simulink model "fundamentalModel"  (R2023a)
settings: Solver=FixedStepAuto  StartTime=0.0  StopTime=1681200  FixedStep=60  RelTol=1e-3
model workspace (MAT data in the model file):
  c1 = Simulink.Parameter
  c1.Value = Simulink.data.Expression
  c1.Value.ExpressionString = " rho_s/rho_m"
  c1.DataType = 'auto'
  c1.Complexity = 'real'
  c1.Dimensions = -1
  c2 = Simulink.Parameter
  c2.Value = Simulink.data.Expression
  c2.Value.ExpressionString = " 1/(rho_m*pi*R^2)"
  c2.DataType = 'auto'
  c2.Complexity = 'real'
  c2.Dimensions = -1
  c3 = Simulink.Parameter
  c3.Value = Simulink.data.Expression
  c3.Value.ExpressionString = " r_m^2*(2*g)^0.5/(R^2)"
  c3.DataType = 'auto'
  c3.Complexity = 'real'
  c3.Dimensions = -1
  c4 = Simulink.Parameter
  c4.Value = Simulink.data.Expression
  c4.Value.ExpressionString = " 1/(rho_m*Cp_matte)"
  c4.DataType = 'auto'
  c4.Complexity = 'real'
  c4.Dimensions = -1
  c5 = Simulink.Parameter
  c5.Value = Simulink.data.Expression
  c5.Value.ExpressionString = " r_s^2*(2*g)^0.5/(R^2)"
  c5.DataType = 'auto'
  c5.Complexity = 'real'
  c5.Dimensions = -1
undefined symbols (not defined in the file or in its folder): a, alpha_Co, alpha_Cu, alpha_Fe, alpha_Ni, b, Cp_bar_eq, Cp_bar_offgas, Cp_bar_slag, Cp_matte, Cp_slag, delta_H_bar_r_coal, delta_H_CoS, delta_H_Cu2S, delta_H_FeS, delta_H_Ni3S2, delta_Ts, epsilon, g, hm_init, hs_hole, m_dot_dust_and_accr, R, r_m, r_s, rho_m, rho_s, sigma, T_amb, T_furnace, Tm_init, U, vFactor_m, vFactor_s
libraries: simulink x3
settings Model: PauseTimes=1.631410e4  PacingRate=1000  Creator=jason.miskin  LastModifiedBy=john.atherfold
settings DataIOCC: ExternalInput=slInputs  LoadExternalInput=on  SaveFormat=Array  InspectSignalLogs=on  OutputOption=AdditionalOutputTimes  OutputTimes=SDO_OutputTimes  ReturnWorkspaceOutputsName=SDOSimTest_Log
settings DebuggingCC: UnconnectedInputMsg=warning  UnconnectedOutputMsg=warning  UnconnectedLineMsg=warning
settings ModelReferenceCC: EnableRefExpFcnMdlSchedulingChecks=on
settings RTWCC: DLArmComputeVersion=19.05

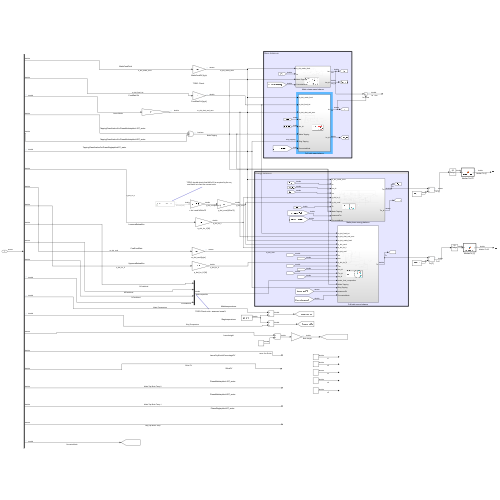
[thumbnail: Simulink's stored preview of the top-level diagram]
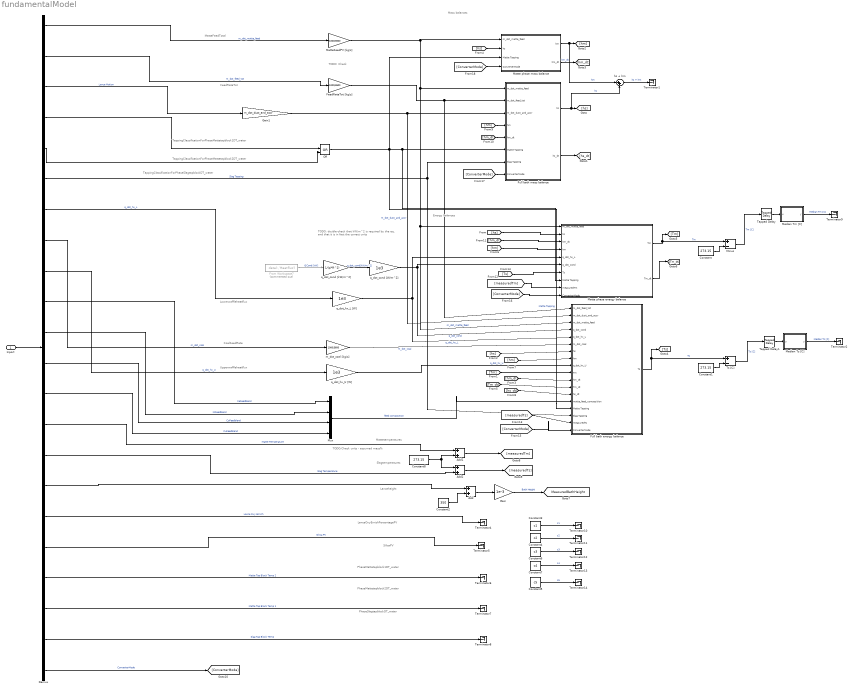
== system fundamentalModel ==
  note: PhaseSlagtapblockDT_water
  note: PhaseMattetapblock2DT_water
  note: PhaseMattetapblock1DT_water
  note: SilicaPV
  note: LanceOxyEnrishPercentagePV
  note: Lanceheight
  note: Slagtemperatures
  note: Mattetemperatures
  note: Upperwaffleheatflux
  note: CoalFeedRate
  note: Lowerwaffleheatflux
  note: TappingClassificationForPhaseSlagtapblockDT_water
  note: TappingClassificationForPhaseMattetapblock2DT_water
  note: TappingClassificationForPhaseMattetapblock1DT_water
  note: FeedRateTot
  note: MatteFeedTotal
  note: TODO: double-check that kW/m^2 is required by the eq,
      |  and that it is in fact the correct units
  note: TODO: Check
  note: TODO:Check units - assumed mass%
  note: Mass balances
  note: Energy balances
  Inport : Inport
  Add : Sum
  Add1 : Sum
  Add2 : Sum
  Constant : Constant  Value=273.15
  Constant1 : Constant  Value=273.15
  Constant2 : Constant  Value=350
  Constant3 : Constant  Value=c1
  Constant4 : Constant  Value=c2
  Constant5 : Constant  Value=c5
  Constant6 : Constant  Value=c3
  Constant7 : Constant  Value=c4
  Constant8 : Constant  Value=273.15
  Demux : Demux  Outputs=22
  "FeedRateTot [kg/s] " : Gain  Gain=1000/3600
  From Workspace7 : FromWorkspace  Commented=on  VariableName=data(:,'Heatflux')  SampleTime=-1
  Full bath energy balance : Subsystem
  Full bath mass balance : Subsystem
  Gain : Gain  Gain=1e-3
  Gain1 : Gain  Gain=m_dot_dust_and_accr
  Matte phase energy balance : Subsystem
  Matte phase mass balance : Subsystem
  MatteFeedPV [kg/s] : Gain  Gain=1000/3600
  Median Tm [C] : MATLAB Function  TreatAsAtomicUnit=on
  Median Ts [C] : MATLAB Function  TreatAsAtomicUnit=on
  Minus : Sum  Inputs=+-
  Mux : Mux
  OR : Logic  Operator=OR  IconShape=distinctive  AllPortsSameDT=off  OutDataTypeStr=boolean
  Tapped Delay : simulink/Discrete/Tapped Delay  vinit=Tm_init - 273.15  samptime=-1  NumDelays=50  DelayOrder=Oldest  includeCurrent=off
  Tapped Delay1 : simulink/Discrete/Tapped Delay  vinit=Tm_init - 273.15  samptime=-1  NumDelays=50  DelayOrder=Oldest  includeCurrent=off
  Terminator{1..2,4..14} (13 alike) : Terminator
  Ts [C] : Sum  Inputs=+-
  hs + hm : Sum  Inputs=|++
  m_dot_coal [kg/s] : Gain  Gain=1000/3600
  q_dot_cond [W/m^2] : Gain  Gain=1e3
  q_dot_cond [kW/m^2] : Gain  Gain=1/(pi*R^2)
  q_dot_hx_L [W] : Gain  Gain=1e3
  q_dot_hx_U [W] : Gain  Gain=1e3
  tag scope: MeasuredBathHeight=global
  wires:
  Inport/1 -> Demux/1
  Matte phase mass balance/1(hm) -> [hm], hs + hm/1  "hm"
  Matte phase mass balance/2(hm_dt) -> [hm_dt]  "hm_dt"
  Demux/2 -> "FeedRateTot [kg/s] "/1  "m_dot_feed_tot"
  Gain1/1 -> Full bath energy balance/2(m_dot_dust_and_accr), Full bath mass balance/3(m_dot_dust_and_accr)  "m_dot_dust_and_accr"
  Full bath mass balance/1(hs) -> hs + hm/2, [hs]  "hs"
  Demux/7 -> q_dot_hx_L [W]/1  "q_dot_hx_L"
  q_dot_cond [W/m^2]/1 -> Matte phase energy balance/6(q_dot_cond), Full bath energy balance/4(q_dot_cond)  "q_dot_cond"
  Full bath energy balance/1(Ts) -> [Ts], Ts [C]/1  "Ts"
  Matte phase energy balance/1(Tm) -> [Tm], Minus/1  "Tm"
  Matte phase energy balance/2(Tm_dt) -> [Tm_dt]
  Full bath mass balance/2(hs_dt) -> [hs_dt]
  [hs] -> Matte phase energy balance/2(hs)
  [hs] -> Matte phase mass balance/2(hs)
  [hm] -> Matte phase energy balance/4(hm)
  [hm] -> Full bath mass balance/4(hm)
  [hm_dt] -> Full bath mass balance/5(hm_dt)
  [hm_dt] -> Matte phase energy balance/3(hm_dt)
  Demux/8 -> m_dot_coal [kg/s]/1  "m_dot_coal"
  [Ts] -> Matte phase energy balance/7(Ts)
  [hs] -> Full bath energy balance/7(hs)
  [hm] -> Full bath energy balance/8(hm)
  Demux/9 -> q_dot_hx_U [W]/1  "q_dot_hx_U"
  [Tm] -> Full bath energy balance/10(Tm)
  [hm_dt] -> Full bath energy balance/11(hm_dt)
  [Tm_dt] -> Full bath energy balance/12(Tm_dt)
  [hs_dt] -> Full bath energy balance/13(hs_dt)
  Mux/1 -> Full bath energy balance/14(matte_feed_composition)  "feed composition"
  MatteFeedPV [kg/s]/1 -> Full bath energy balance/3(m_dot_matte_feed), Matte phase energy balance/1(m_dot_matte_feed), Full bath mass balance/1(m_dot_matte_feed), Matte phase mass balance/1(m_dot_matte_feed)  "m_dot_matte_feed"
  "FeedRateTot [kg/s] "/1 -> Full bath energy balance/1(m_dot_feed_tot), Full bath mass balance/2(m_dot_feed_tot)
  Demux/10 -> Mux/1  "FeFeedblend"
  Demux/11 -> Mux/2  "NiFeedblend"
  Demux/12 -> Mux/3  "CoFeedblend"
  Demux/13 -> Mux/4  "CuFeedblend"
  From Workspace7/1 -> q_dot_cond [kW/m^2]/1  "QCond [kW]"
  q_dot_hx_U [W]/1 -> Full bath energy balance/9(q_dot_hx_U)  "q_dot_hx_U"
  q_dot_hx_L [W]/1 -> Full bath energy balance/5(q_dot_hx_L), Matte phase energy balance/5(q_dot_hx_L)  "q_dot_hx_L"
  Demux/14 -> Add1/1  "Matte Temperature"
  m_dot_coal [kg/s]/1 -> Full bath energy balance/6(m_dot_coal)  "m_dot_coal"
  hs + hm/1 -> Terminator1/1  "hs + hm"
  q_dot_cond [kW/m^2]/1 -> q_dot_cond [W/m^2]/1  "q_dot_cond[kW/m^2]"
  Minus/1 -> Tapped Delay/1  "Tm [C]"
  Constant/1 -> Minus/2
  Constant1/1 -> Ts [C]/2
  Ts [C]/1 -> Tapped Delay1/1  "Ts [C]"
  Demux/16 -> Add/1
  Gain/1 -> [MeasuredBathHeight]  "Bath Height"
  Add/1 -> Gain/1
  Constant2/1 -> Add/2
  Demux/4 -> OR/1
  Demux/5 -> OR/2
  OR/1 -> Full bath energy balance/15(Matte Tapping), Matte phase energy balance/8(Matte Tapping), Full bath mass balance/6(Matte Tapping), Matte phase mass balance/3(Matte Tapping)  "Matte Tapping"
  Demux/6 -> Full bath mass balance/7(Slag Tapping), Full bath energy balance/16(Slag Tapping)  "Slag Tapping"
  Demux/17 -> Terminator4/1  "Lance Oxy Enrich"
  Demux/18 -> Terminator5/1  "Silica PV"
  Demux/19 -> Terminator6/1  "Matte Tap Block Temp 2"
  Demux/20 -> Terminator7/1  "Matte Tap Block Temp 1"
  Demux/21 -> Terminator8/1  "Slag Tap Block Temp"
  Demux/15 -> Add2/2  "Slag Temperature"
  Tapped Delay/1 -> Median Tm [C]/1(u)
  Median Tm [C]/1(y) -> Terminator9/1  "Median Tm [C]"
  Constant3/1 -> Terminator10/1  "c1"
  Constant5/1 -> Terminator14/1  "c5"
  Constant7/1 -> Terminator13/1  "c4"
  Constant6/1 -> Terminator12/1  "c3"
  Constant4/1 -> Terminator11/1  "c2"
  Demux/1 -> MatteFeedPV [kg/s]/1  "m_dot_matte_feed"
  Tapped Delay1/1 -> Median Ts [C]/1(u)
  Median Ts [C]/1(y) -> Terminator2/1  "Median Ts [C]"
  Demux/3 -> Gain1/1  "Lance Motion"
  [measuredTm] -> Matte phase energy balance/9(measuredTm)
  [measuredTs] -> Full bath energy balance/17(measuredTs)
  Constant8/1 -> Add2/1, Add1/2
  Add1/1 -> [measuredTm]
  Add2/1 -> [measuredTs]
  Demux/22 -> [ConverterMode]  "ConverterMode"
  [ConverterMode] -> Matte phase energy balance/10(ConverterMode)
  [ConverterMode] -> Full bath energy balance/18(ConverterMode)
  [ConverterMode] -> Matte phase mass balance/4(ConverterMode)
  [ConverterMode] -> Full bath mass balance/8(ConverterMode)

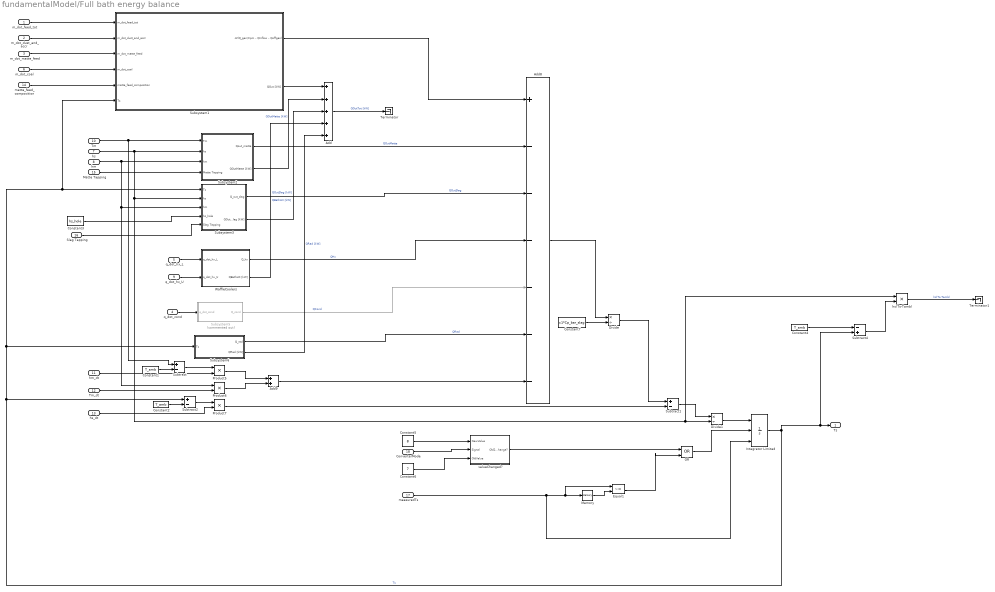
== system fundamentalModel/Full bath energy balance ==
  m_dot_feed_tot : Inport
  m_dot_dust_and_accr : Inport  Port=2
  m_dot_matte_feed : Inport  Port=3
  q_dot_cond : Inport  Port=4
  q_dot_hx_L : Inport  Port=5
  m_dot_coal : Inport  Port=6
  hs : Inport  Port=7
  hm : Inport  Port=8
  q_dot_hx_U : Inport  Port=9
  Tm : Inport  Port=10
  hm_dt : Inport  Port=11
  Tm_dt : Inport  Port=12
  hs_dt : Inport  Port=13
  matte_feed_composition : Inport  Port=14
  Matte Tapping : Inport  Port=15
  Slag Tapping : Inport  Port=16
  measuredTs : Inport  Port=17
  ConverterMode : Inport  Port=18
  Add : Sum  Inputs=+++++
  Add8 : Sum  Inputs=+------
  Add9 : Sum
  Constant1 : Constant  Value=T_amb
  Constant2 : Constant  Value=T_amb
  Constant3 : Constant  Value=hs_hole
  Constant4 : Constant  Value=T_amb
  Constant5 : Constant  Value=8
  Constant6 : Constant  Value=7
  Constant7 : Constant  Value=c1*Cp_bar_slag
  Divide : Product  Inputs=*/
  Divide1 : Product  Inputs=*/
  Equal1 : RelationalOperator  Operator=~=  OutDataTypeStr=boolean  RndMeth=Simplest  InputSameDT=off
  Integrator Limited : Integrator  ExternalReset=rising  InitialConditionSource=external  LimitOutput=on  LowerSaturationLimit=T_amb
  Memory : Memory
  OR : Logic  Operator=OR  IconShape=distinctive  AllPortsSameDT=off  OutDataTypeStr=boolean
  Product5 : Product
  Product6 : Product
  Product7 : Product
  Subsystem1 : Subsystem
  Subsystem2 : Subsystem
  Subsystem3 : Subsystem
  Subsystem5 : Subsystem  Commented=on
  Subsystem6 : Subsystem
  Subtract : Sum  Inputs=+-
  Subtract1 : Sum  Inputs=+-
  Subtract2 : Sum  Inputs=+-
  Subtract4 : Sum  Inputs=-+
  Terminator : Terminator
  Terminator1 : Terminator
  WaffleCoolers : Subsystem
  hs(Ts-Tamb) : Product  Inputs=**
  valueChanged? : Subsystem
  Ts : Outport
  wires:
  q_dot_cond/1 -> Subsystem5/1(q_dot_cond)
  Divide1/1 -> Integrator Limited/1
  matte_feed_composition/1 -> Subsystem1/5(matte_feed_composition)
  m_dot_feed_tot/1 -> Subsystem1/1(m_dot_feed_tot)
  Add8/1 -> Divide/1
  m_dot_dust_and_accr/1 -> Subsystem1/2(m_dot_dust_and_accr)
  Divide/1 -> Subtract1/1
  m_dot_coal/1 -> Subsystem1/4(m_dot_coal)
  m_dot_matte_feed/1 -> Subsystem1/3(m_dot_matte_feed)
  WaffleCoolers/1(Q_hx) -> Add8/4  "QHx"
  Subsystem3/1(Q_out_slag) -> Add8/3  "QOutSlag"
  Tm_dt/1 -> Product6/2
  hs/1 -> hs(Ts-Tamb)/1, Divide1/2, Subsystem3/2(hs), Subsystem2/2(hs)
  hm_dt/1 -> Product5/2
  q_dot_hx_U/1 -> WaffleCoolers/2(q_dot_hx_U)
  q_dot_hx_L/1 -> WaffleCoolers/1(q_dot_hx_L)
  Subsystem5/1(Q_cond) -> Add8/5  "QCond"
  Product5/1 -> Add9/1
  Constant7/1 -> Divide/2
  Product6/1 -> Add9/2
  Tm/1 -> Subtract/1, Subsystem2/1(Tm)
  Subsystem1/1(c2(Q_gen/Cpm - Qinflow - Qoffgas)) -> Add8/1
  Subsystem2/1(Qout_matte) -> Add8/2  "QOutMatte"
  hs_dt/1 -> Product7/2
  Product7/1 -> Subtract1/2
  Add9/1 -> Add8/7
  Constant3/1 -> Subsystem3/4(hs_hole)
  Subtract1/1 -> Divide1/1
  Subsystem6/1(Q_rad) -> Add8/6  "QRad"
  hm/1 -> Product6/1, Subsystem3/3(hm), Subsystem2/3(hm)
  Integrator Limited/1 -> Subtract4/2, Ts/1, Subtract2/1, Subsystem6/1(Ts), Subsystem1/6(Ts), Subsystem3/1(Ts)  "Ts"
  Matte Tapping/1 -> Subsystem2/4(Matte Tapping)
  Slag Tapping/1 -> Subsystem3/5(Slag Tapping)
  Subsystem1/2(QOut [kW]) -> Add/1
  Subsystem2/2(QOutMatte [kW]) -> Add/2  "QOutMatte [kW]"
  Subsystem3/2(QOutSlag [kW]) -> Add/3  "QOutSlag [kW]"
  WaffleCoolers/2(QBathHX [kW]) -> Add/4  "QBathHX [kW]"
  Subsystem6/2(QRad [kW]) -> Add/5  "QRad [kW]"
  Add/1 -> Terminator/1  "QOutTot [kW]"
  Subtract/1 -> Product5/1
  Constant1/1 -> Subtract/2
  Constant2/1 -> Subtract2/2
  Subtract2/1 -> Product7/1
  hs(Ts-Tamb)/1 -> Terminator1/1  "hs(Ts-Tamb)"
  Constant4/1 -> Subtract4/1
  Subtract4/1 -> hs(Ts-Tamb)/2
  Memory/1 -> Equal1/2
  ConverterMode/1 -> valueChanged?/2(Signal)
  Constant5/1 -> valueChanged?/1(NewValue)
  valueChanged?/1(Old2NewChange?) -> OR/1
  measuredTs/1 -> Equal1/1, Memory/1, Integrator Limited/3
  Constant6/1 -> valueChanged?/3(OldValue)
  OR/1 -> Integrator Limited/2
  Equal1/1 -> OR/2

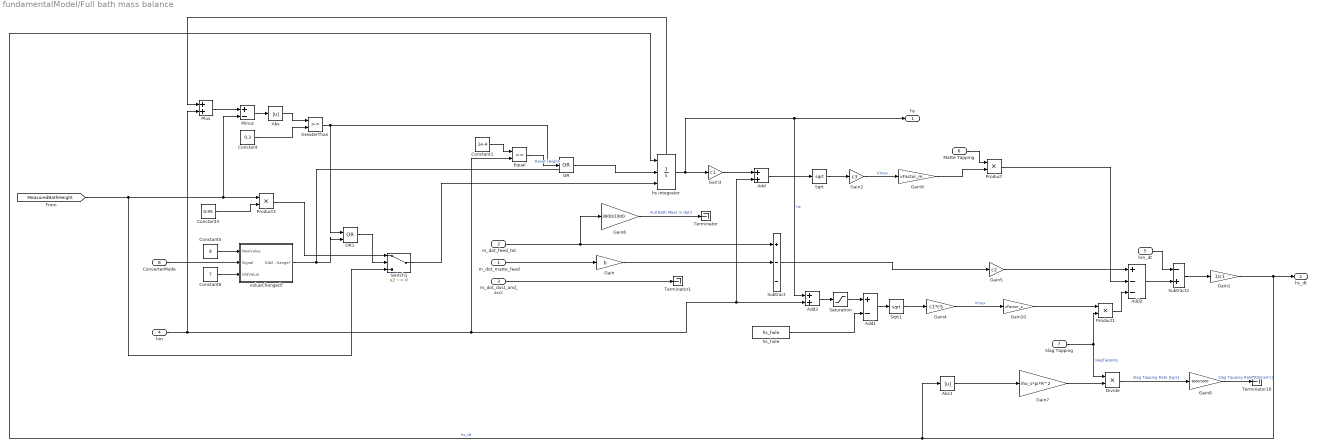
== system fundamentalModel/Full bath mass balance ==
  m_dot_matte_feed : Inport
  m_dot_feed_tot : Inport  Port=2
  m_dot_dust_and_accr : Inport  Port=3
  hm : Inport  Port=4
  hm_dt : Inport  Port=5
  Matte Tapping : Inport  Port=6
  Slag Tapping : Inport  Port=7
  ConverterMode : Inport  Port=8
  Abs : Abs  SaturateOnIntegerOverflow=off
  Abs1 : Abs  SaturateOnIntegerOverflow=off
  Add : Sum
  Add1 : Sum  Inputs=+-
  Add2 : Sum  Inputs=+--
  Add3 : Sum
  Constant : Constant  Value=0.3
  Constant1 : Constant  Value=1e-4
  Constant3 : Constant  Value=0.95
  Constant5 : Constant  Value=8
  Constant6 : Constant  Value=7
  Divide : Product  Inputs=**
  Equal : RelationalOperator  Operator===  OutDataTypeStr=boolean  RndMeth=Simplest  InputSameDT=off
  Gain : Gain  Gain=b
  Gain1 : Gain  Gain=1/c1
  Gain10 : Gain  Gain=vFactor_s
  Gain2 : Gain  Gain=c3
  Gain3 : Gain  Gain=c1
  Gain4 : Gain  Gain=c1*c5
  Gain5 : Gain  Gain=c2
  Gain6 : Gain  Gain=3600/1000
  Gain7 : Gain  Gain=rho_s*pi*R^2
  Gain8 : Gain  Gain=3600/1000
  Gain9 : Gain  Gain=vFactor_m
  GreaterThan : RelationalOperator  OutDataTypeStr=boolean  RndMeth=Simplest  InputSameDT=off
  Minus : Sum  Inputs=+-
  OR : Logic  Operator=OR  Inputs=3  IconShape=distinctive  AllPortsSameDT=off  OutDataTypeStr=boolean
  OR1 : Logic  Operator=OR  IconShape=distinctive  AllPortsSameDT=off  OutDataTypeStr=boolean
  Plus : Sum
  Product : Product
  Product1 : Product
  Product3 : Product
  Saturation : Saturate  UpperLimit=inf  LowerLimit=hs_hole
  Sqrt : Sqrt
  Sqrt1 : Sqrt  OutputSignalType=real
  Subtract : Sum  Inputs=+--
  Subtract2 : Sum  Inputs=-+
  Switch1 : Switch  Criteria=u2 ~= 0  SaturateOnIntegerOverflow=off  InputSameDT=off
  Terminator : Terminator
  Terminator1 : Terminator
  Terminator10 : Terminator
  hs integrator : Integrator  ExternalReset=level hold  InitialConditionSource=external  InitialCondition=1  LimitOutput=on  LowerSaturationLimit=hs_hole  ShowStatePort=on
  hs_hole : Constant  Value=hs_hole
  valueChanged? : Subsystem
  hs : Outport
  hs_dt : Outport  Port=2
  wires:
  Sqrt1/1 -> Gain4/1
  Gain5/1 -> Add2/1
  Gain/1 -> Subtract/2
  Add2/1 -> Subtract2/2
  Subtract/1 -> Gain5/1
  Gain1/1 -> hs_dt/1, Abs1/1, hs integrator/1  "hs_dt"
  m_dot_dust_and_accr/1 -> Terminator1/1
  Gain3/1 -> Add/1
  Add1/1 -> Sqrt1/1
  Add/1 -> Sqrt/1
  m_dot_feed_tot/1 -> Gain6/1, Subtract/1
  hm/1 -> Plus/2, Add3/2, Add/2, Equal/2
  Subtract2/1 -> Gain1/1
  Sqrt/1 -> Gain2/1
  hm_dt/1 -> Subtract2/1
  hs integrator/1 -> hs/1, Add3/1, Gain3/1  "hs"
  m_dot_matte_feed/1 -> Gain/1
  Product/1 -> Add2/2
  Product1/1 -> Add2/3
  Slag Tapping/1 -> Product1/2, Divide/1  "slagTapping"
  Gain6/1 -> Terminator/1  "Full Bath Mass in (tph)"
  Matte Tapping/1 -> Product/1
  hs_hole/1 -> Add1/2
  Add3/1 -> Saturation/1
  Saturation/1 -> Add1/1
  Constant1/1 -> Equal/1
  Equal/1 -> OR/2  "Reset Height"
  Divide/1 -> Gain8/1  "Slag Tapping Rate [kg/s]"
  Gain7/1 -> Divide/2
  Abs1/1 -> Gain7/1
  Gain8/1 -> Terminator10/1  "Slag Tapping Rate [tonne/hr]"
  Gain2/1 -> Gain9/1  "Vmax"
  Gain9/1 -> Product/2
  Gain4/1 -> Gain10/1  "Vmax"
  Gain10/1 -> Product1/1
  ConverterMode/1 -> valueChanged?/2(Signal)
  valueChanged?/1(Old2NewChange?) -> OR/3, OR1/2
  Switch1/1 -> hs integrator/3
  [MeasuredBathHeight] -> Switch1/3, Minus/2, Product3/1
  Constant3/1 -> Product3/2
  Constant5/1 -> valueChanged?/1(NewValue)
  Constant6/1 -> valueChanged?/3(OldValue)
  OR/1 -> hs integrator/2
  Product3/1 -> Switch1/1
  Plus/1 -> Minus/1
  Constant/1 -> GreaterThan/2
  Minus/1 -> Abs/1
  Abs/1 -> GreaterThan/1
  GreaterThan/1 -> OR1/1, OR/1
  OR1/1 -> Switch1/2
  hs integrator/State -> Plus/1

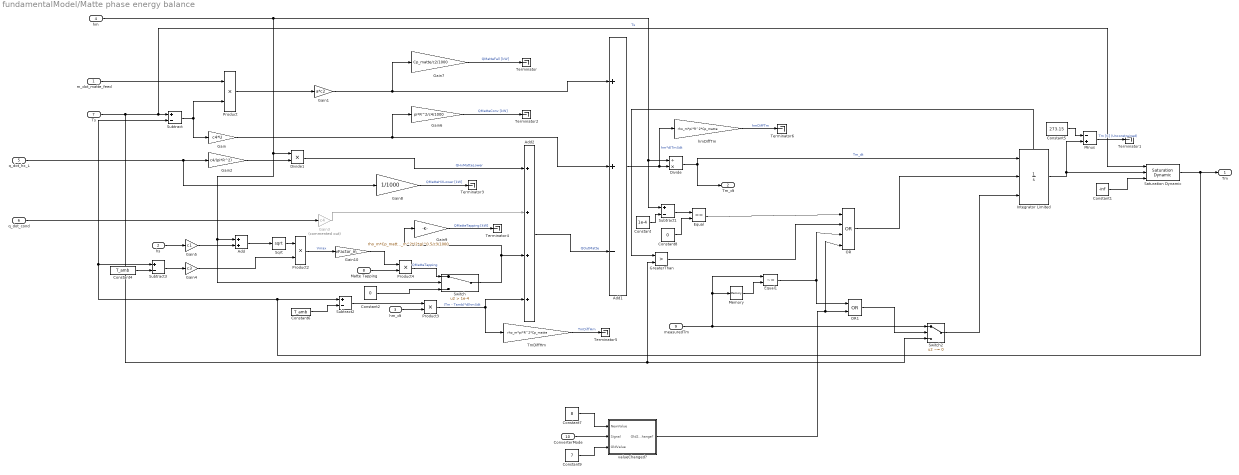
== system fundamentalModel/Matte phase energy balance ==
  m_dot_matte_feed : Inport
  hs : Inport  Port=2
  hm_dt : Inport  Port=3
  hm : Inport  Port=4
  q_dot_hx_L : Inport  Port=5
  q_dot_cond : Inport  Port=6
  Ts : Inport  Port=7
  Matte Tapping : Inport  Port=8
  measuredTm : Inport  Port=9
  ConverterMode : Inport  Port=10
  Add : Sum
  Add1 : Sum  Inputs=++-
  Add2 : Sum  Inputs=++++
  Constant : Constant  Value=1e-4
  Constant1 : Constant  Value=-inf
  Constant2 : Constant  Value=0
  Constant4 : Constant  Value=T_amb
  Constant5 : Constant  Value=273.15
  Constant6 : Constant  Value=T_amb
  Constant7 : Constant  Value=8
  Constant8 : Constant  Value=0
  Constant9 : Constant  Value=7
  Divide : Product  Inputs=/*
  Divide1 : Product  Inputs=**
  Equal : RelationalOperator  Operator===  OutDataTypeStr=boolean  RndMeth=Simplest  InputSameDT=off
  Equal1 : RelationalOperator  Operator=~=  OutDataTypeStr=boolean  RndMeth=Simplest  InputSameDT=off
  Gain : Gain  Gain=c4*U
  Gain1 : Gain  Gain=a*c2
  Gain10 : Gain  Gain=vFactor_m
  Gain2 : Gain  Gain=c4/(pi*R^2)
  Gain3 : Gain  Commented=on  Gain=c4
  Gain4 : Gain  Gain=c3
  Gain5 : Gain  Gain=c1
  Gain6 : Gain  Gain=pi*R^2/c4/1000
  Gain7 : Gain  Gain=Cp_matte/c2/1000
  Gain8 : Gain  Gain=1/1000
  Gain9 : Gain  Gain=rho_m*Cp_matte*pi*r_m^2*(2*g)^0.5/c3/1000
  GreaterThan : RelationalOperator  Operator=>  OutDataTypeStr=boolean  RndMeth=Simplest  InputSameDT=off
  Integrator Limited : Integrator  ExternalReset=level hold  InitialConditionSource=external  LimitOutput=on  LowerSaturationLimit=T_amb  ShowStatePort=on
  Memory : Memory
  Minus : Sum  Inputs=-+
  OR : Logic  Operator=OR  Inputs=4  IconShape=distinctive  AllPortsSameDT=off  OutDataTypeStr=boolean
  OR1 : Logic  Operator=OR  IconShape=distinctive  AllPortsSameDT=off  OutDataTypeStr=boolean
  Product{,2..4} (4 alike) : Product
  Saturation Dynamic : simulink/Discontinuities/Saturation Dynamic  OutMin=[]  OutMax=[]  OutDataTypeStr=Inherit: Same as second input  OutDataType=fixdt(1, 16)  OutScaling=2^-10  DoSatur=off
  Sqrt : Sqrt
  Subtract{,1..3} (4 alike) : Sum  Inputs=+-
  Switch : Switch  Criteria=u2 > Threshold  Threshold=1e-4  SaturateOnIntegerOverflow=off  InputSameDT=off
  Switch2 : Switch  Criteria=u2 ~= 0  Threshold=1  SaturateOnIntegerOverflow=off  InputSameDT=off
  Terminator{,1..6} (7 alike) : Terminator
  TmDiffHm : Gain  Gain=rho_m*pi*R^2*Cp_matte
  hmDiffTm : Gain  Gain=rho_m*pi*R^2*Cp_matte
  valueChanged? : Subsystem
  Tm : Outport
  Tm_dt : Outport  Port=2
  wires:
  Add/1 -> Sqrt/1
  hm/1 -> Divide1/1, Switch/2, Add/1, Divide/1, Subtract1/1
  Add1/1 -> hmDiffTm/1, Divide/2  "hm*d(Tm)/dt"
  hm_dt/1 -> Product3/2
  Subtract/1 -> Gain/1, Product/2
  Sqrt/1 -> Product2/1
  m_dot_matte_feed/1 -> Product/1
  Gain3/1 -> Add2/2
  Gain4/1 -> Product2/2
  Product/1 -> Gain1/1
  Gain5/1 -> Add/2
  q_dot_hx_L/1 -> Gain8/1, Gain2/1
  Gain/1 -> Gain6/1, Add1/2
  Ts/1 -> Saturation Dynamic/1, Subtract/1, GreaterThan/2, Switch2/3  "Ts"
  Divide1/1 -> Add2/1  "QHxMatteLower"
  Divide/1 -> Tm_dt/1, Integrator Limited/1  "Tm_dt"
  hs/1 -> Gain5/1
  q_dot_cond/1 -> Gain3/1
  Product4/1 -> Switch/1  "QMatteTapping"
  Matte Tapping/1 -> Product4/2
  Product3/1 -> TmDiffHm/1, Add2/4  "(Tm - Tamb)*d(hm)/dt"
  Add2/1 -> Add1/3  "QOutMatte"
  Gain6/1 -> Terminator2/1  "QMatteConv [kW]"
  Gain7/1 -> Terminator/1  "QMatteFall [kW]"
  Gain8/1 -> Terminator3/1  "QMatteHXLower [kW]"
  Constant1/1 -> Saturation Dynamic/3
  Gain9/1 -> Terminator4/1  "QMatteTapping [kW]"
  Constant2/1 -> Switch/3
  Switch/1 -> Add2/3, Gain9/1
  Subtract1/1 -> Equal/1
  Constant/1 -> Subtract1/2
  Constant4/1 -> Subtract3/2
  Subtract3/1 -> Gain4/1
  TmDiffHm/1 -> Terminator5/1  "TmDiffHm"
  hmDiffTm/1 -> Terminator6/1  "hmDiffTm"
  Gain1/1 -> Gain7/1, Add1/1
  Integrator Limited/1 -> Minus/2, Saturation Dynamic/2
  Constant5/1 -> Minus/1
  Minus/1 -> Terminator1/1  "Tm [C] (Unconstrained)"
  Subtract2/1 -> Product3/1
  Constant6/1 -> Subtract2/2
  Saturation Dynamic/1 -> Tm/1, Subtract/2, Subtract3/1, Subtract2/1
  Constant8/1 -> Equal/2
  Equal/1 -> OR/1
  OR/1 -> Integrator Limited/2
  GreaterThan/1 -> OR/2
  Integrator Limited/State -> GreaterThan/1
  Gain2/1 -> Divide1/2
  Memory/1 -> Equal1/2
  Equal1/1 -> OR1/1, OR/3
  Switch2/1 -> Integrator Limited/3
  Product2/1 -> Gain10/1  "Vmax"
  Gain10/1 -> Product4/1
  valueChanged?/1(Old2NewChange?) -> OR/4, OR1/2
  measuredTm/1 -> Equal1/1, Memory/1, Switch2/1
  OR1/1 -> Switch2/2
  ConverterMode/1 -> valueChanged?/2(Signal)
  Constant7/1 -> valueChanged?/1(NewValue)
  Constant9/1 -> valueChanged?/3(OldValue)

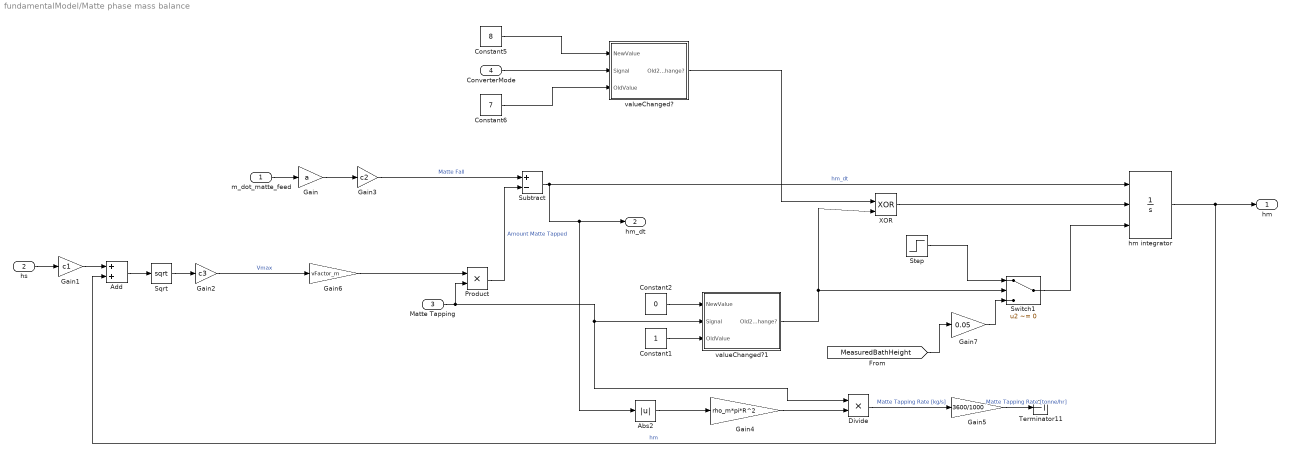
== system fundamentalModel/Matte phase mass balance ==
  m_dot_matte_feed : Inport
  hs : Inport  Port=2
  Matte Tapping : Inport  Port=3
  ConverterMode : Inport  Port=4
  Abs2 : Abs  SaturateOnIntegerOverflow=off
  Add : Sum
  Constant1 : Constant
  Constant2 : Constant  Value=0
  Constant5 : Constant  Value=8
  Constant6 : Constant  Value=7
  Divide : Product  Inputs=**
  Gain : Gain  Gain=a
  Gain1 : Gain  Gain=c1
  Gain2 : Gain  Gain=c3
  Gain3 : Gain  Gain=c2
  Gain4 : Gain  Gain=rho_m*pi*R^2
  Gain5 : Gain  Gain=3600/1000
  Gain6 : Gain  Gain=vFactor_m
  Gain7 : Gain  Gain=0.05
  Product : Product
  Sqrt : Sqrt
  Step : Step  Before=hm_init  After=1e-4  SampleTime=0
  Subtract : Sum  Inputs=+-
  Switch1 : Switch  Criteria=u2 ~= 0  SaturateOnIntegerOverflow=off  InputSameDT=off
  Terminator11 : Terminator
  XOR : Logic  Operator=XOR  IconShape=distinctive  AllPortsSameDT=off  OutDataTypeStr=boolean
  hm integrator : Integrator  ExternalReset=rising  InitialConditionSource=external  InitialCondition=hm_init  LimitOutput=on  LowerSaturationLimit=1e-4
  valueChanged? : Subsystem
  valueChanged?1 : Subsystem
  hm : Outport
  hm_dt : Outport  Port=2
  wires:
  Add/1 -> Sqrt/1
  Sqrt/1 -> Gain2/1
  hm integrator/1 -> Add/2, hm/1  "hm"
  m_dot_matte_feed/1 -> Gain/1
  hs/1 -> Gain1/1
  Gain/1 -> Gain3/1
  Gain1/1 -> Add/1
  Product/1 -> Subtract/2  "Amount Matte Tapped"
  Gain3/1 -> Subtract/1  "Matte Fall"
  Subtract/1 -> Abs2/1, hm_dt/1, hm integrator/1  "hm_dt"
  Divide/1 -> Gain5/1  "Matte Tapping Rate [kg/s]"
  Abs2/1 -> Gain4/1
  Gain4/1 -> Divide/2
  Gain5/1 -> Terminator11/1  "Matte Tapping Rate [tonne/hr]"
  Gain2/1 -> Gain6/1  "Vmax"
  Gain6/1 -> Product/1
  Switch1/1 -> hm integrator/3
  Step/1 -> Switch1/1
  [MeasuredBathHeight] -> Gain7/1
  Gain7/1 -> Switch1/3
  XOR/1 -> hm integrator/2
  Constant1/1 -> valueChanged?1/3(OldValue)
  Matte Tapping/1 -> valueChanged?1/2(Signal), Divide/1, Product/2
  Constant2/1 -> valueChanged?1/1(NewValue)
  valueChanged?1/1(Old2NewChange?) -> Switch1/2, XOR/2
  Constant5/1 -> valueChanged?/1(NewValue)
  ConverterMode/1 -> valueChanged?/2(Signal)
  Constant6/1 -> valueChanged?/3(OldValue)
  valueChanged?/1(Old2NewChange?) -> XOR/1

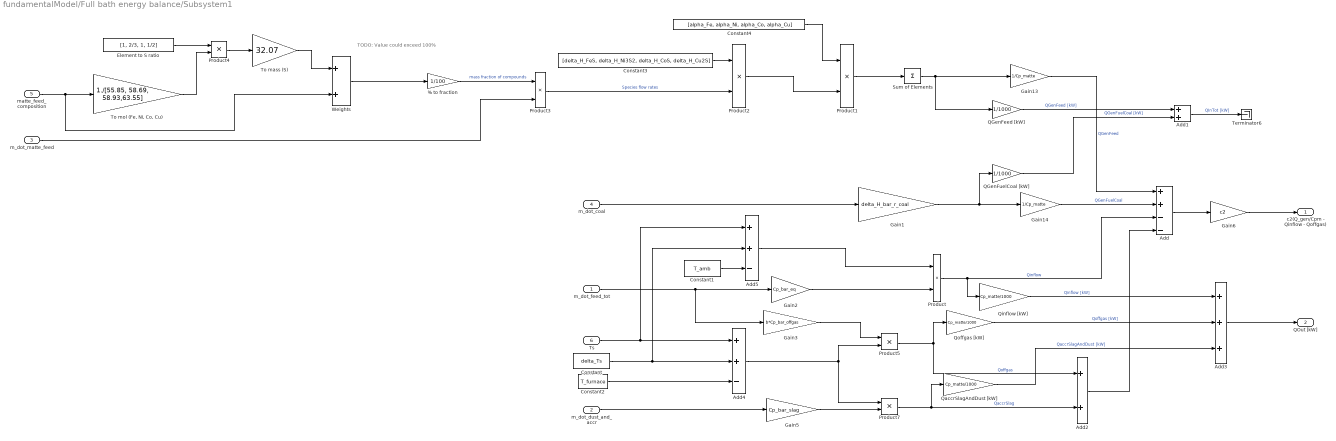
== system fundamentalModel/Full bath energy balance/Subsystem1 ==
  note: TODO: Value could exceed 100%
  m_dot_feed_tot : Inport
  m_dot_dust_and_accr : Inport  Port=2
  m_dot_matte_feed : Inport  Port=3
  m_dot_coal : Inport  Port=4
  matte_feed_composition : Inport  Port=5
  Ts : Inport  Port=6
  % to fraction : Gain  Gain=1/100
  Add : Sum  Inputs=++--
  Add1 : Sum
  Add2 : Sum
  Add3 : Sum  Inputs=+++
  Add4 : Sum  Inputs=++-
  Add5 : Sum  Inputs=++-
  Constant : Constant  Value=delta_Ts
  Constant1 : Constant  Value=T_amb
  Constant2 : Constant  Value=T_furnace
  Constant3 : Constant  Value=[delta_H_FeS, delta_H_Ni3S2, delta_H_CoS, delta_H_Cu2S]
  Constant4 : Constant  Value=[alpha_Fe, alpha_Ni, alpha_Co, alpha_Cu]
  Element to S ratio : Constant  Value=[1, 2/3, 1, 1/2]
  Gain1 : Gain  Gain=delta_H_bar_r_coal
  Gain13 : Gain  Gain=1/Cp_matte
  Gain14 : Gain  Gain=1/Cp_matte
  Gain2 : Gain  Gain=Cp_bar_eq
  Gain3 : Gain  Gain=b*Cp_bar_offgas
  Gain5 : Gain  Gain=Cp_bar_slag
  Gain6 : Gain  Gain=c2
  Product{,1..5,7} (7 alike) : Product
  QGenFeed [kW] : Gain  Gain=1/1000
  QGenFuelCoal [kW] : Gain  Gain=1/1000
  QaccrSlagAndDust [kW] : Gain  Gain=Cp_matte/1000
  Qinflow [kW] : Gain  Gain=Cp_matte/1000
  Qoffgas [kW] : Gain  Gain=Cp_matte/1000
  Sum of Elements : Sum  Inputs=+
  Terminator6 : Terminator
  To mass (S) : Gain  Gain=32.07
  "To mol (Fe, Ni, Co, Cu)" : Gain  Gain=1./[55.85, 58.69, 58.93,63.55]
  Weights : Sum
  c2(Q_gen/Cpm - Qinflow - Qoffgas) : Outport
  QOut [kW] : Outport  Port=2
  wires:
  Add2/1 -> Add/4
  m_dot_feed_tot/1 -> Gain3/1, Gain2/1
  Gain5/1 -> Product7/2
  Gain3/1 -> Product5/1
  Add4/1 -> Product7/1, Product5/2
  Add/1 -> Gain6/1
  Gain1/1 -> QGenFuelCoal [kW]/1, Gain14/1
  Gain2/1 -> Product/2
  m_dot_coal/1 -> Gain1/1
  Product/1 -> Qinflow [kW]/1, Add/3  "Qinflow"
  Gain6/1 -> c2(Q_gen/Cpm - Qinflow - Qoffgas)/1
  Constant/1 -> Add5/2, Add4/2
  Constant3/1 -> Product2/1
  m_dot_matte_feed/1 -> Product3/2
  Product3/1 -> Product2/2  "Species flow rates"
  matte_feed_composition/1 -> Weights/2, "To mol (Fe, Ni, Co, Cu)"/1
  Product4/1 -> To mass (S)/1
  Element to S ratio/1 -> Product4/1
  To mass (S)/1 -> Weights/1
  "To mol (Fe, Ni, Co, Cu)"/1 -> Product4/2
  Weights/1 -> % to fraction/1
  % to fraction/1 -> Product3/1  "mass fraction of compounds"
  Constant1/1 -> Add5/3
  Ts/1 -> Add5/1, Add4/1
  Product7/1 -> Add2/2, QaccrSlagAndDust [kW]/1  "QaccrSlag"
  Product5/1 -> Qoffgas [kW]/1, Add2/1  "Qoffgas"
  QGenFeed [kW]/1 -> Add1/1  "QGenFeed [kW]"
  QGenFuelCoal [kW]/1 -> Add1/2  "QGenFuelCoal [kW]"
  Qinflow [kW]/1 -> Add3/1  "Qinflow [kW]"
  Qoffgas [kW]/1 -> Add3/2  "Qoffgas [kW]"
  QaccrSlagAndDust [kW]/1 -> Add3/3  "QaccrSlagAndDust [kW]"
  Add1/1 -> Terminator6/1  "QInTot [kW]"
  Add3/1 -> QOut [kW]/1
  Gain13/1 -> Add/1  "QGenFeed"
  Gain14/1 -> Add/2  "QGenFuelCoal"
  m_dot_dust_and_accr/1 -> Gain5/1
  Constant2/1 -> Add4/3
  Add5/1 -> Product/1
  Sum of Elements/1 -> QGenFeed [kW]/1, Gain13/1
  Product1/1 -> Sum of Elements/1
  Product2/1 -> Product1/2
  Constant4/1 -> Product1/1

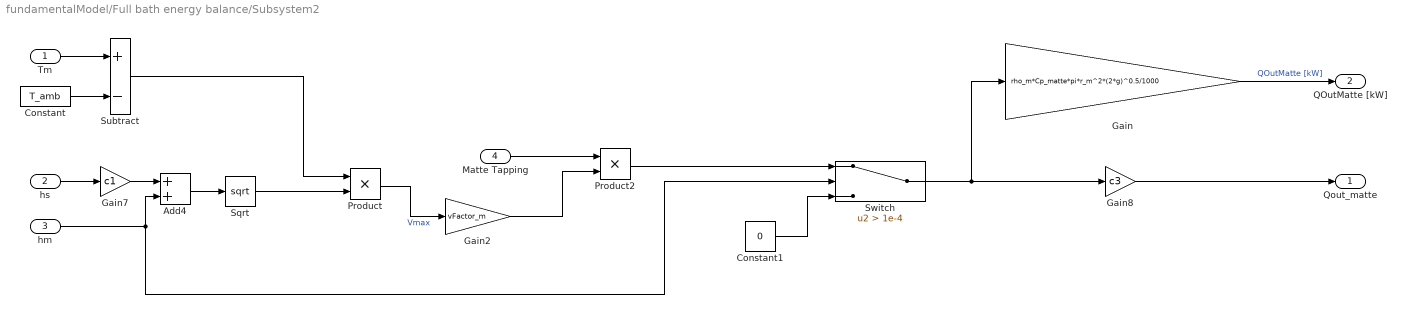
== system fundamentalModel/Full bath energy balance/Subsystem2 ==
  Tm : Inport
  hs : Inport  Port=2
  hm : Inport  Port=3
  Matte Tapping : Inport  Port=4
  Add4 : Sum
  Constant : Constant  Value=T_amb
  Constant1 : Constant  Value=0
  Gain : Gain  Gain=rho_m*Cp_matte*pi*r_m^2*(2*g)^0.5/1000
  Gain2 : Gain  Gain=vFactor_m
  Gain7 : Gain  Gain=c1
  Gain8 : Gain  Gain=c3
  Product : Product
  Product2 : Product
  Sqrt : Sqrt
  Subtract : Sum  Inputs=+-
  Switch : Switch  Criteria=u2 > Threshold  Threshold=1e-4  SaturateOnIntegerOverflow=off  InputSameDT=off
  Qout_matte : Outport
  QOutMatte [kW] : Outport  Port=2
  wires:
  Gain7/1 -> Add4/1
  Add4/1 -> Sqrt/1
  Tm/1 -> Subtract/1
  hm/1 -> Switch/2, Add4/2
  hs/1 -> Gain7/1
  Matte Tapping/1 -> Product2/1
  Sqrt/1 -> Product/2
  Product2/1 -> Switch/1
  Gain/1 -> QOutMatte [kW]/1  "QOutMatte [kW]"
  Switch/1 -> Gain/1, Gain8/1
  Constant1/1 -> Switch/3
  Constant/1 -> Subtract/2
  Subtract/1 -> Product/1
  Gain8/1 -> Qout_matte/1
  Product/1 -> Gain2/1  "Vmax"
  Gain2/1 -> Product2/2

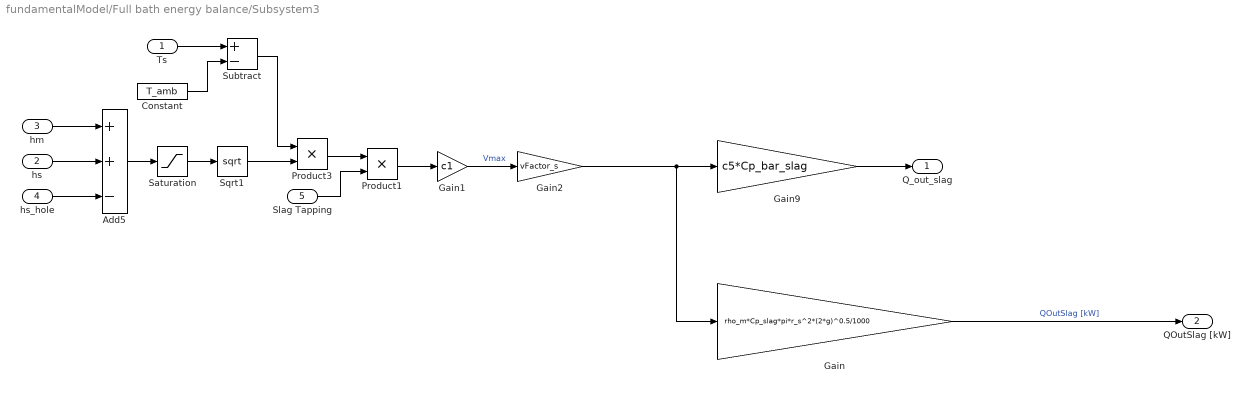
== system fundamentalModel/Full bath energy balance/Subsystem3 ==
  Ts : Inport
  hs : Inport  Port=2
  hm : Inport  Port=3
  hs_hole : Inport  Port=4
  Slag Tapping : Inport  Port=5
  Add5 : Sum  Inputs=++-
  Constant : Constant  Value=T_amb
  Gain : Gain  Gain=rho_m*Cp_slag*pi*r_s^2*(2*g)^0.5/1000
  Gain1 : Gain  Gain=c1
  Gain2 : Gain  Gain=vFactor_s
  Gain9 : Gain  Gain=c5*Cp_bar_slag
  Product1 : Product
  Product3 : Product
  Saturation : Saturate  UpperLimit=inf  LowerLimit=0
  Sqrt1 : Sqrt  OutputSignalType=real
  Subtract : Sum  Inputs=+-
  Q_out_slag : Outport
  QOutSlag [kW] : Outport  Port=2
  wires:
  Sqrt1/1 -> Product3/2
  Gain9/1 -> Q_out_slag/1
  hs/1 -> Add5/2
  Product3/1 -> Product1/1
  hm/1 -> Add5/1
  hs_hole/1 -> Add5/3
  Add5/1 -> Saturation/1
  Ts/1 -> Subtract/1
  Slag Tapping/1 -> Product1/2
  Product1/1 -> Gain1/1
  Saturation/1 -> Sqrt1/1
  Gain/1 -> QOutSlag [kW]/1  "QOutSlag [kW]"
  Constant/1 -> Subtract/2
  Subtract/1 -> Product3/1
  Gain1/1 -> Gain2/1  "Vmax"
  Gain2/1 -> Gain/1, Gain9/1

== system fundamentalModel/Full bath energy balance/Subsystem5 ==
  q_dot_cond : Inport
  Gain12 : Gain  Gain=c4
  Q_cond : Outport
  wires:
  q_dot_cond/1 -> Gain12/1
  Gain12/1 -> Q_cond/1

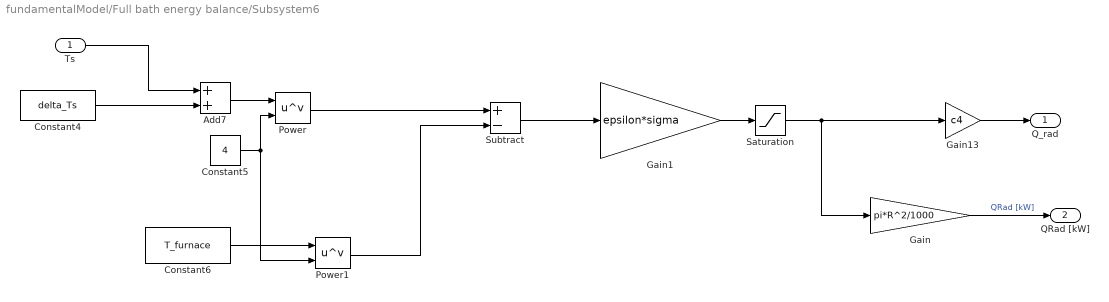
== system fundamentalModel/Full bath energy balance/Subsystem6 ==
  Ts : Inport
  Add7 : Sum
  Constant4 : Constant  Value=delta_Ts
  Constant5 : Constant  Value=4
  Constant6 : Constant  Value=T_furnace
  Gain : Gain  Gain=pi*R^2/1000
  Gain1 : Gain  Gain=epsilon*sigma
  Gain13 : Gain  Gain=c4
  Power : Math  Operator=pow
  Power1 : Math  Operator=pow
  Saturation : Saturate  UpperLimit=inf  LowerLimit=0
  Subtract : Sum  Inputs=+-
  Q_rad : Outport
  QRad [kW] : Outport  Port=2
  wires:
  Subtract/1 -> Gain1/1
  Power/1 -> Subtract/1
  Constant5/1 -> Power1/2, Power/2
  Constant6/1 -> Power1/1
  Add7/1 -> Power/1
  Power1/1 -> Subtract/2
  Constant4/1 -> Add7/2
  Ts/1 -> Add7/1
  Gain13/1 -> Q_rad/1
  Gain1/1 -> Saturation/1
  Gain/1 -> QRad [kW]/1  "QRad [kW]"
  Saturation/1 -> Gain/1, Gain13/1

== system fundamentalModel/Full bath energy balance/WaffleCoolers ==
  q_dot_hx_L : Inport
  q_dot_hx_U : Inport  Port=2
  Add6 : Sum
  Gain : Gain  Gain=1/1000
  Gain1 : Gain  Gain=c4/(pi*R^2)
  Q_hx : Outport
  QBathHX [kW] : Outport  Port=2
  wires:
  Gain1/1 -> Q_hx/1  "QBathHX [nonD]"
  q_dot_hx_L/1 -> Add6/1
  q_dot_hx_U/1 -> Add6/2
  Gain/1 -> QBathHX [kW]/1  "QBathHX [kW]"
  Add6/1 -> Gain/1, Gain1/1

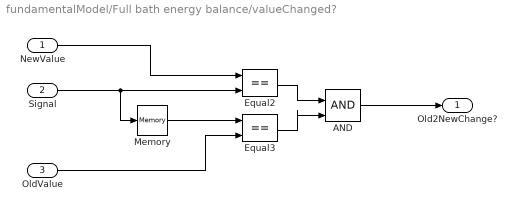
== system fundamentalModel/Full bath energy balance/valueChanged? ==
  NewValue : Inport
  Signal : Inport  Port=2
  OldValue : Inport  Port=3
  AND : Logic  IconShape=distinctive  AllPortsSameDT=off  OutDataTypeStr=boolean
  Equal2 : RelationalOperator  Operator===  OutDataTypeStr=boolean  RndMeth=Simplest  InputSameDT=off
  Equal3 : RelationalOperator  Operator===  OutDataTypeStr=boolean  RndMeth=Simplest  InputSameDT=off
  Memory : Memory  InheritSampleTime=on
  Old2NewChange? : Outport
  wires:
  AND/1 -> Old2NewChange?/1
  Signal/1 -> Equal2/2, Memory/1
  Equal2/1 -> AND/1
  OldValue/1 -> Equal3/2
  Equal3/1 -> AND/2
  Memory/1 -> Equal3/1
  NewValue/1 -> Equal2/1

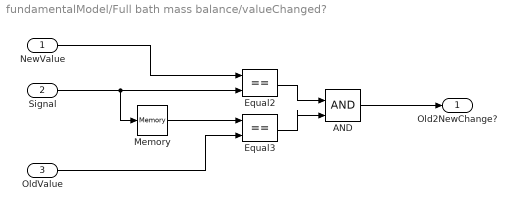
== system fundamentalModel/Full bath mass balance/valueChanged? ==
  NewValue : Inport
  Signal : Inport  Port=2
  OldValue : Inport  Port=3
  AND : Logic  IconShape=distinctive  AllPortsSameDT=off  OutDataTypeStr=boolean
  Equal2 : RelationalOperator  Operator===  OutDataTypeStr=boolean  RndMeth=Simplest  InputSameDT=off
  Equal3 : RelationalOperator  Operator===  OutDataTypeStr=boolean  RndMeth=Simplest  InputSameDT=off
  Memory : Memory  InheritSampleTime=on
  Old2NewChange? : Outport
  wires:
  AND/1 -> Old2NewChange?/1
  Signal/1 -> Equal2/2, Memory/1
  Equal2/1 -> AND/1
  OldValue/1 -> Equal3/2
  Equal3/1 -> AND/2
  Memory/1 -> Equal3/1
  NewValue/1 -> Equal2/1

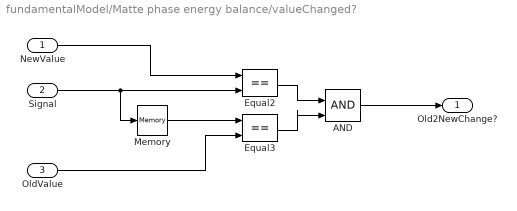
== system fundamentalModel/Matte phase energy balance/valueChanged? ==
  NewValue : Inport
  Signal : Inport  Port=2
  OldValue : Inport  Port=3
  AND : Logic  IconShape=distinctive  AllPortsSameDT=off  OutDataTypeStr=boolean
  Equal2 : RelationalOperator  Operator===  OutDataTypeStr=boolean  RndMeth=Simplest  InputSameDT=off
  Equal3 : RelationalOperator  Operator===  OutDataTypeStr=boolean  RndMeth=Simplest  InputSameDT=off
  Memory : Memory  InheritSampleTime=on
  Old2NewChange? : Outport
  wires:
  AND/1 -> Old2NewChange?/1
  Signal/1 -> Equal2/2, Memory/1
  Equal2/1 -> AND/1
  OldValue/1 -> Equal3/2
  Equal3/1 -> AND/2
  Memory/1 -> Equal3/1
  NewValue/1 -> Equal2/1

== system fundamentalModel/Matte phase mass balance/valueChanged? ==
  NewValue : Inport
  Signal : Inport  Port=2
  OldValue : Inport  Port=3
  AND : Logic  IconShape=distinctive  AllPortsSameDT=off  OutDataTypeStr=boolean
  Equal2 : RelationalOperator  Operator===  OutDataTypeStr=boolean  RndMeth=Simplest  InputSameDT=off
  Equal3 : RelationalOperator  Operator===  OutDataTypeStr=boolean  RndMeth=Simplest  InputSameDT=off
  Memory : Memory  InheritSampleTime=on
  Old2NewChange? : Outport
  wires:
  AND/1 -> Old2NewChange?/1
  Signal/1 -> Equal2/2, Memory/1
  Equal2/1 -> AND/1
  OldValue/1 -> Equal3/2
  Equal3/1 -> AND/2
  Memory/1 -> Equal3/1
  NewValue/1 -> Equal2/1

== system fundamentalModel/Matte phase mass balance/valueChanged?1 ==
  NewValue : Inport
  Signal : Inport  Port=2
  OldValue : Inport  Port=3
  AND : Logic  IconShape=distinctive  AllPortsSameDT=off  OutDataTypeStr=boolean
  Equal2 : RelationalOperator  Operator===  OutDataTypeStr=boolean  RndMeth=Simplest  InputSameDT=off
  Equal3 : RelationalOperator  Operator===  OutDataTypeStr=boolean  RndMeth=Simplest  InputSameDT=off
  Memory : Memory  InheritSampleTime=on
  Old2NewChange? : Outport
  wires:
  AND/1 -> Old2NewChange?/1
  Signal/1 -> Equal2/2, Memory/1
  Equal2/1 -> AND/1
  OldValue/1 -> Equal3/2
  Equal3/1 -> AND/2
  Memory/1 -> Equal3/1
  NewValue/1 -> Equal2/1

== matlab function fundamentalModel/Median Tm [C] ==
  data: u input; y output
function y = simMedian(u)
%% Median Function - used to implement a moving median in Simulink
y = median(u);
end

== matlab function fundamentalModel/Median Ts [C] ==
  data: u input; y output
function y = simMedian(u)
%% Median Function - used to implement a moving median in Simulink
y = median(u);
end
